simulink model "s2"  (Simulink 7.4)
settings: Solver=ode45  StartTime=0.0  StopTime=5  RelTol=1e-3
libraries: dspsrcs4 x2, dspsigops x1, dsparch4 x1, dspsnks4 x1
settings Model: Creator=ml43519  LastModifiedBy=ml43519  SimulationMode=accelerator

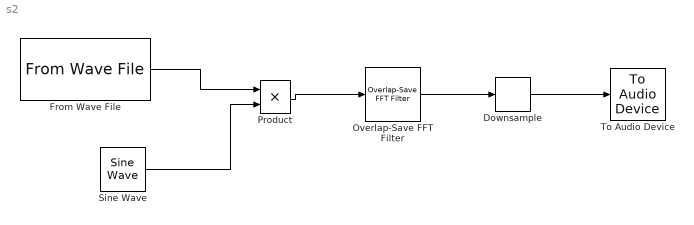
== system s2 ==
  Downsample : dspsigops/Downsample  N=4  phase=0  ic=0  smode=Allow multirate  fmode=Maintain input frame size
  From Wave File : dspsrcs4/From Wave File  FileName=0036435195.wav  SamplesPerFrame=1024  MinBufSize=1024  dType=double  bLoop=off  timesToPlay=1  restartMode=immediately after last sample  firstSampleOutput=off  lastSampleOutput=off
  Overlap-Save FFT Filter : dsparch4/Overlap-Save FFT Filter  SystemSampleTime=-1  nfft_in=2048  h=4*fir1(64,0.1)  output_complexity=Real
  Product : Product  OutDataType=fixdt(1, 16)  OutScaling=2^0  RndMeth=Zero
  Sine Wave : dspsrcs4/Sine Wave  Amplitude=0.5  Frequency=60000  Phase=pi/2  SampleMode=Discrete  OutComplex=Real  CompMethod=Trigonometric fcn  TableSize=Speed  SampleTime=1/176400  SamplesPerFrame=1024  dataType=double  wordLen=16  udDataType=sfix(16)  fracBitsMode=Best precision  numFracBits=15  ResetState=Restart at time zero
  To Audio Device : dspsnks4/To Audio Device  DialogController=dspDDGCreate  DialogControllerArgs=DataTag0  deviceName=Default  inheritSampleRate=on  sampleRate=44100  deviceDatatype=Determine from input data type  autoBufferSize=on  bufferSize=4096  queueDuration=1.0
  wires:
  Sine Wave/1 -> Product/2
  From Wave File/1 -> Product/1
  Product/1 -> Overlap-Save FFT Filter/1
  Overlap-Save FFT Filter/1 -> Downsample/1
  Downsample/1 -> To Audio Device/1
